simulink library "subsystems"  (R2024b)
settings: Solver=VariableStepAuto  StartTime=0.0  StopTime=10.0  RelTol=1e-3
libraries: fl_lib x2, nesl_utility x2
settings Model: Creator=Nicholas Quillin  LastModifiedBy=Nicholas Quillin

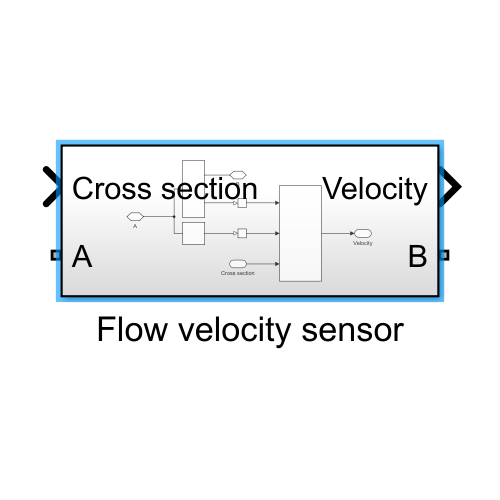
[thumbnail: Simulink's stored preview of the top-level diagram]
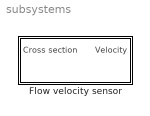
== system subsystems ==
  Flow velocity sensor : Subsystem

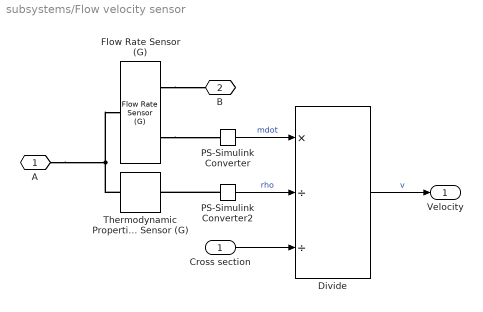
== system subsystems/Flow velocity sensor ==
  Cross section : Inport
  Divide : Product  Inputs=*//
  Flow Rate Sensor (G) : fl_lib/Gas/Sensors/Flow Rate Sensor (G)  mass_flow_measure=true  volumetric_flow_measure=false  volumetric_flow_conditions=foundation.enum.volumetric_flow_conditions.actual  p_std=0.101325 MPa  T_std=20 degC  energy_flow_measure=false
      settings: InternalSimscapePortConfiguration="{\"Bottom\":[],\"Left\":[{\"id\":\"A\",\"label\":\"A\",\"type\":\"foundation.gas.gas\"}],\"Right\":[{\"id\":\"B\",\"label\":\"B\",\"type\":\"foundation.gas.gas\"},{\"id\":\"M\",\"label\":\"M\",\"type\":\"output\"}],\"Top\":[]}"
  PS-Simulink Converter : nesl_utility/PS-Simulink Converter  PhysicalDomain=network_engine_domain  SubClassName=ps_output  LeftPortType=input  RightPortType=output  PseudoPeriodic=off  Frequencies=[]  VectorFormat=inherit  Unit=kg/s  AffineConversion=off
  PS-Simulink Converter2 : nesl_utility/PS-Simulink Converter  PhysicalDomain=network_engine_domain  SubClassName=ps_output  LeftPortType=input  RightPortType=output  PseudoPeriodic=off  Frequencies=[]  VectorFormat=inherit  Unit=kg/m^3  AffineConversion=off
  Thermodynamic Properties Sensor (G) : fl_lib/Gas/Sensors/Thermodynamic Properties Sensor (G)  enthalpy=false  density=true  specific_heat=false  entropy=false  s_std=3.8635 kJ/(K*kg)  p_std=0.101325 MPa  T_std=293.15 K
      settings: InternalSimscapePortConfiguration="{\"Bottom\":[],\"Left\":[{\"id\":\"A\",\"label\":\"A\",\"type\":\"foundation.gas.gas\"}],\"Right\":[{\"id\":\"RHO\",\"label\":\"ρ\",\"type\":\"output\"}],\"Top\":[]}"
  A : PMIOPort  Side=Left
  B : PMIOPort  Port=2  Side=Right
  Velocity : Outport
  wires:
  Cross section/1 -> Divide/3
  PS-Simulink Converter/1 -> Divide/1  "mdot"
  PS-Simulink Converter2/1 -> Divide/2  "rho"
  Divide/1 -> Velocity/1  "v"
  connections:
  PS-Simulink Converter2/LConn1 -- Thermodynamic Properties Sensor (G)/RConn1
  Thermodynamic Properties Sensor (G)/LConn1 -- Flow Rate Sensor (G)/LConn1 -- A/RConn1
  Flow Rate Sensor (G)/RConn2 -- PS-Simulink Converter/LConn1
  Flow Rate Sensor (G)/RConn1 -- B/RConn1
